simulink model "Pulse24Rectifier"  (R2023b)
settings: Solver=VariableStepAuto  StartTime=0.0  StopTime=0.1  RelTol=1e-3
undefined symbols (not defined in the file or in its folder): D1, D11, Delta
libraries: spsCurrentMeasurementLib x26, spsDiodeLib x24, spsVoltageMeasurementLib x4, spsACVoltageSourceLib x3, spsThreePhaseTransformerThreeWindingsLib x2, spsGroundLib x1, spsSeriesRLCBranchLib x1, spsZigzagPhaseShiftingTransformerLib x1, spspowerguiLib x1
settings Model: Creator=HP  LastModifiedBy=HP
settings SolverCC: ZeroCrossAlgorithm=Adaptive
settings DataIOCC: Refine=10
settings DebuggingCC: IgnoredZcDiagnostic=none

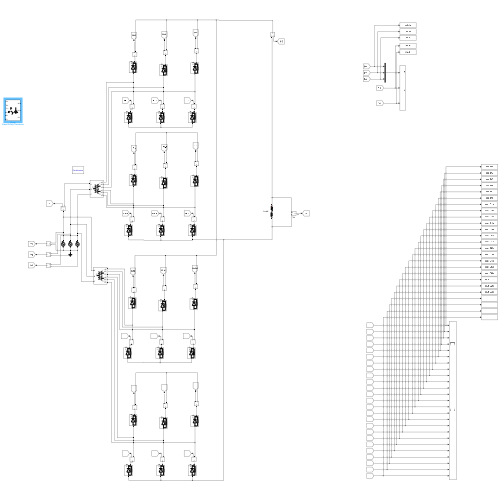
[thumbnail: Simulink's stored preview of the top-level diagram]
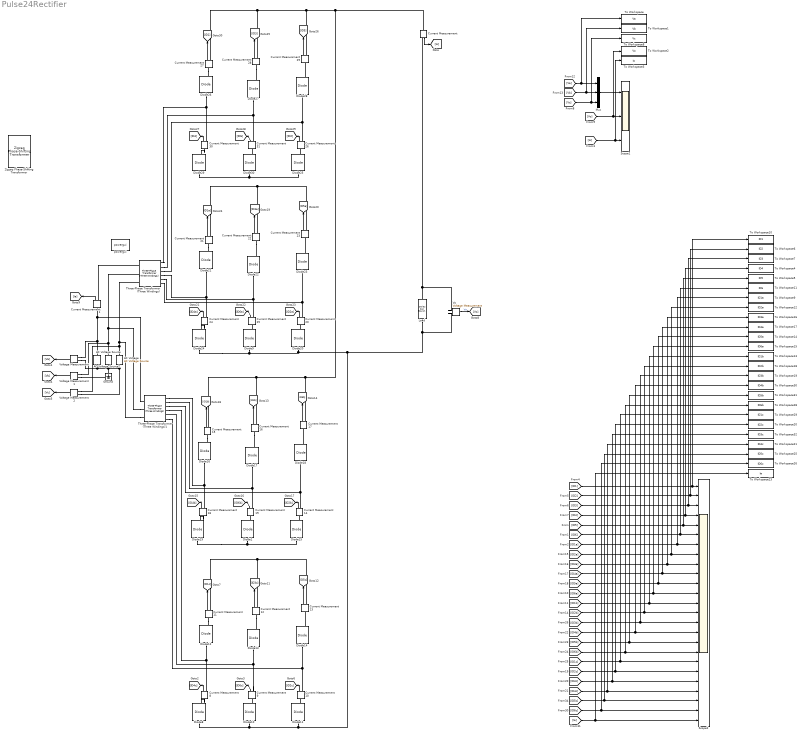
== system Pulse24Rectifier ==
  AC Voltage : spsACVoltageSourceLib/AC Voltage Source  Amplitude=480*sqrt(2)/sqrt(3)  Phase=120  Frequency=60  SampleTime=0  Measurements=None  BusType=swing  Pref=10e3  Qref=0  Qmin=-inf  Qmax=+inf
  AC Voltage Source : spsACVoltageSourceLib/AC Voltage Source  Amplitude=480*sqrt(2)/sqrt(3)  Phase=-120  Frequency=60  SampleTime=0  Measurements=None  BusType=swing  Pref=10e3  Qref=0  Qmin=-inf  Qmax=+inf
  AC Voltage Source2 : spsACVoltageSourceLib/AC Voltage Source  Amplitude=480*sqrt(2)/sqrt(3)  Phase=0  Frequency=60  SampleTime=0  Measurements=None  BusType=swing  Pref=10e3  Qref=0  Qmin=-inf  Qmax=+inf
  Current Measurement{,1,8..31} (26 alike) : spsCurrentMeasurementLib/Current Measurement  PhasorSimulation=off  OutputType=Complex  PSBequivalent=0
  Diode{1,8..30} (24 alike) : spsDiodeLib/Diode  Ron=0.001  Lon=0  Vf=0.8  IC=0  UseSnubber=0  Rs=500  Cs=250e-9  Measurements=on
  Ground : spsGroundLib/Ground  LConnTagsString=a
  Load : spsSeriesRLCBranchLib/Series RLC Branch  LConnTagsString=__new0  RConnTagsString=__new0  BranchType=RL  Resistance=11.08  Inductance=0.0224  SetiL0=off  InitialCurrent=0  Capacitance=1e-6  Setx0=off  InitialVoltage=0  Measurements=None
  Mux : Mux  Inputs=3
  Scope1 : Scope  NumInputPorts=3
  Scope2 : Scope  NumInputPorts=25
  Three-Phase Transformer (Three Windings) : spsThreePhaseTransformerThreeWindingsLib/Three-Phase Transformer (Three Windings)  Winding1Connection=Delta (D1)  Winding2Connection=Y  Winding3Connection=Delta (D11)  CoreType=Three single-phase transformers  SetSaturation=off  Hysteresis=off  DataFile='hysteresis'  SetInitialFlux=off  Measurements=None  UNITS=pu  NominalPower=[ 250e3 , 50 ]  Winding1=[ 300 , 0.002 , 0.08 ]  Winding2=[ 100 , 0.002 , 0.08 ]  Winding3=[ 100 , 0.002 , 0.08 ]  Rm=500  Lm=500  L0=0.5  Saturation=[ 0,0 ; 0.0024,1.2 ; 1.0,1.52 ]  InitialFluxes=[0.8 -0.8 0.7]  BreakLoop=off  DiscreteSolver=Trapezoidal iterative  DataType=off  TransfoNumber=1
      settings: LibrarySourceBlock=|
      | sps_lib/Power Grid Elements/Three-Phase
      | Transformer
      | (Three Windings)
  Three-Phase Transformer (Three Windings)1 : spsThreePhaseTransformerThreeWindingsLib/Three-Phase Transformer (Three Windings)  Winding1Connection=Delta (D1)  Winding2Connection=Y  Winding3Connection=Delta (D11)  CoreType=Three single-phase transformers  SetSaturation=off  Hysteresis=off  DataFile='hysteresis'  SetInitialFlux=off  Measurements=None  UNITS=pu  NominalPower=[ 250e3 , 50 ]  Winding1=[ 300 , 0.002 , 0.08 ]  Winding2=[ 100 , 0.002 , 0.08 ]  Winding3=[ 100 , 0.002 , 0.08 ]  Rm=500  Lm=500  L0=0.5  Saturation=[ 0,0 ; 0.0024,1.2 ; 1.0,1.52 ]  InitialFluxes=[0.8 -0.8 0.7]  BreakLoop=off  DiscreteSolver=Trapezoidal iterative  DataType=off  TransfoNumber=1
      settings: LibrarySourceBlock=|
      | sps_lib/Power Grid Elements/Three-Phase
      | Transformer
      | (Three Windings)
  To Workspace : ToWorkspace  VariableName=Va  SaveFormat=Timeseries  SampleTime=-1
  To Workspace1 : ToWorkspace  VariableName=Vb  SaveFormat=Timeseries  SampleTime=-1
  To Workspace10 : ToWorkspace  VariableName=ID1  SaveFormat=Timeseries  SampleTime=-1
  To Workspace11 : ToWorkspace  VariableName=ID6  SaveFormat=Timeseries  SampleTime=-1
  To Workspace12 : ToWorkspace  VariableName=ID2a  SaveFormat=Timeseries  SampleTime=-1
  To Workspace13 : ToWorkspace  VariableName=ID1b  SaveFormat=Timeseries  SampleTime=-1
  To Workspace14 : ToWorkspace  VariableName=ID5a  SaveFormat=Timeseries  SampleTime=-1
  To Workspace15 : ToWorkspace  VariableName=ID6a  SaveFormat=Timeseries  SampleTime=-1
  To Workspace16 : ToWorkspace  VariableName=ID3a  SaveFormat=Timeseries  SampleTime=-1
  To Workspace17 : ToWorkspace  VariableName=ID4a  SaveFormat=Timeseries  SampleTime=-1
  To Workspace18 : ToWorkspace  VariableName=ID2b  SaveFormat=Timeseries  SampleTime=-1
  To Workspace19 : ToWorkspace  VariableName=ID3b  SaveFormat=Timeseries  SampleTime=-1
  To Workspace2 : ToWorkspace  VariableName=Vo  SaveFormat=Timeseries  SampleTime=-1
  To Workspace20 : ToWorkspace  VariableName=ID2c  SaveFormat=Timeseries  SampleTime=-1
  To Workspace21 : ToWorkspace  VariableName=ID4c  SaveFormat=Timeseries  SampleTime=-1
  To Workspace23 : ToWorkspace  VariableName=Ia  SaveFormat=Timeseries  SampleTime=-1
  To Workspace25 : ToWorkspace  VariableName=ID5c  SaveFormat=Timeseries  SampleTime=-1
  To Workspace26 : ToWorkspace  VariableName=ID6c  SaveFormat=Timeseries  SampleTime=-1
  To Workspace28 : ToWorkspace  VariableName=ID6b  SaveFormat=Timeseries  SampleTime=-1
  To Workspace29 : ToWorkspace  VariableName=ID1c  SaveFormat=Timeseries  SampleTime=-1
  To Workspace3 : ToWorkspace  VariableName=Io  SaveFormat=Timeseries  SampleTime=-1
  To Workspace30 : ToWorkspace  VariableName=ID4b  SaveFormat=Timeseries  SampleTime=-1
  To Workspace31 : ToWorkspace  VariableName=ID5b  SaveFormat=Timeseries  SampleTime=-1
  To Workspace32 : ToWorkspace  VariableName=ID3c  SaveFormat=Timeseries  SampleTime=-1
  To Workspace4 : ToWorkspace  VariableName=ID4  SaveFormat=Timeseries  SampleTime=-1
  To Workspace5 : ToWorkspace  VariableName=ID5  SaveFormat=Timeseries  SampleTime=-1
  To Workspace6 : ToWorkspace  VariableName=ID2  SaveFormat=Timeseries  SampleTime=-1
  To Workspace7 : ToWorkspace  VariableName=ID3  SaveFormat=Timeseries  SampleTime=-1
  To Workspace8 : ToWorkspace  VariableName=Vc  SaveFormat=Timeseries  SampleTime=-1
  To Workspace9 : ToWorkspace  VariableName=ID1a  SaveFormat=Timeseries  SampleTime=-1
  Vo : spsVoltageMeasurementLib/Voltage Measurement  PhasorSimulation=off  OutputType=Complex  PSBequivalent=0
  Voltage Measurement : spsVoltageMeasurementLib/Voltage Measurement  PhasorSimulation=off  OutputType=Complex  PSBequivalent=0
  Voltage Measurement1 : spsVoltageMeasurementLib/Voltage Measurement  PhasorSimulation=off  OutputType=Complex  PSBequivalent=0
  Voltage Measurement2 : spsVoltageMeasurementLib/Voltage Measurement  PhasorSimulation=off  OutputType=Complex  PSBequivalent=0
  Zigzag Phase-Shifting Transformer : spsZigzagPhaseShiftingTransformerLib/Zigzag Phase-Shifting Transformer  SecondaryConnection=Yg  SetSaturation=off  SetInitialFlux=off  Measurements=None  UNITS=pu  NominalPower=[ 100e6 60]  PrimaryVoltage=10e3  SecondaryVoltage="[ 30e3  +15]"  Winding1=[ 0.002 0.08 ]  Winding2="[ 0.002  0.08 ]"  Winding3=[ 0.002 0.08 ]  RmLm=[ 500 500 ]  Rm=500  Saturation=[ 0,0 ; 0.0024,1.2 ; 1.0,1.52 ]  InitialFluxes=[0,0,0]  BreakLoop=off  DiscreteSolver=Trapezoidal iterative  DataType=off
      settings: LibrarySourceBlock=|
      | sps_lib/Power Grid Elements/Zigzag
      | Phase-Shifting Transformer
  powergui : spspowerguiLib/powergui  Priority=1  SimulationMode=Continuous  SampleTime=50e-6  frequency=60  Iterations=50  frequencyindice=60  Pbase=100e6  ErrMax=1e-4  UnitsV=kV  UnitsW=MW  buscounter=0  FunctionMessages=off  echomessages=off  EnableUseOfTLC=off  CurrentSourceSwitches=off  DisableSnubberDevices=off  DisableRonSwitches=off  DisableVfSwitches=off  DisplayEquations=off  AutomaticDiscreteSolvers=off  SolverType=Tustin/Backward Euler (TBE)  Interpol=off  ExternalGateDelay=off  methode=off  Ts=0  x0status=blocks  SPID=off  SwTol=0  HookPort=off  NonlinearTolerance=1e-4  nMaxIteration=100  ContinueOnMaxIteration=off  RestoreLinks=warning  ResistiveCurrentMeasurement=off  Frange=[0:2:500]  Ylog=off  Xlog=on  ShowGrid=off  save=off  variable=ZData  structure=0  ZoomFFT=on  StartTime=0.0  cycles=1  DisplayStyle=1  fundamental=60  FreqAxis=off  MaxFrequency=1000  frequencyindicesteady=1  RmsSteady=1  display=off
  wires:
  Vo/1 -> [Vo]  "Vo"
  Current Measurement8/1 -> [ID4c]
  Current Measurement9/1 -> [ID6c]
  Current Measurement10/1 -> [ID2c]
  Current Measurement11/1 -> [ID1c]
  Current Measurement12/1 -> [ID3c]
  Current Measurement13/1 -> [ID5c]
  Current Measurement17/1 -> [ID5b]
  Current Measurement16/1 -> [ID3b]
  Current Measurement15/1 -> [ID1b]
  Current Measurement14/1 -> [ID2b]
  Current Measurement19/1 -> [ID6b]
  Current Measurement18/1 -> [ID4b]
  Current Measurement24/1 -> [ID4a]
  Current Measurement25/1 -> [ID6a]
  Current Measurement20/1 -> [ID2a]
  Current Measurement21/1 -> [ID1a]
  Current Measurement22/1 -> [ID3a]
  Current Measurement23/1 -> [ID5a]
  Current Measurement29/1 -> [ID5]
  Current Measurement28/1 -> [ID3]
  Current Measurement27/1 -> [ID1]
  Current Measurement26/1 -> [ID2]
  Current Measurement31/1 -> [ID6]
  Current Measurement30/1 -> [ID4]
  Current Measurement/1 -> [Io]
  Voltage Measurement1/1 -> [Vb]
  Voltage Measurement/1 -> [Va]
  Voltage Measurement2/1 -> [Vc]
  [ID4] -> To Workspace4/1, Scope2/4
  [ID6] -> Scope2/6, To Workspace11/1
  [ID1] -> To Workspace10/1, Scope2/1
  [Io] -> To Workspace3/1, Scope1/3
  [Vo] -> To Workspace2/1, Scope1/2
  Mux/1 -> Scope1/1
  [ID5] -> Scope2/5, To Workspace5/1
  [ID2] -> To Workspace6/1, Scope2/2
  [ID3] -> To Workspace7/1, Scope2/3
  [Vc] -> To Workspace8/1, Mux/3
  [Va] -> To Workspace/1, Mux/1
  [ID1a] -> Scope2/7, To Workspace9/1
  [Vb] -> To Workspace1/1, Mux/2
  [Ia] -> To Workspace23/1, Scope2/25
  [ID6c] -> To Workspace26/1, Scope2/24
  [ID5c] -> To Workspace25/1, Scope2/23
  [ID4c] -> To Workspace21/1, Scope2/22
  Current Measurement1/1 -> [Ia]
  [ID2a] -> To Workspace12/1, Scope2/8
  [ID3a] -> To Workspace16/1, Scope2/9
  [ID4a] -> To Workspace17/1, Scope2/10
  [ID5a] -> To Workspace14/1, Scope2/11
  [ID6a] -> To Workspace15/1, Scope2/12
  [ID1b] -> To Workspace13/1, Scope2/13
  [ID2b] -> To Workspace18/1, Scope2/14
  [ID3b] -> To Workspace19/1, Scope2/15
  [ID4b] -> To Workspace30/1, Scope2/16
  [ID5b] -> To Workspace31/1, Scope2/17
  [ID6b] -> To Workspace28/1, Scope2/18
  [ID1c] -> To Workspace29/1, Scope2/19
  [ID2c] -> To Workspace20/1, Scope2/20
  [ID3c] -> To Workspace32/1, Scope2/21
  connections:
  Three-Phase Transformer (Three Windings)1/LConn1 -- AC Voltage Source2/RConn1 -- Voltage Measurement/LConn1 -- Current Measurement1/LConn1
  Three-Phase Transformer (Three Windings)1/LConn2 -- AC Voltage Source/RConn1 -- Voltage Measurement1/LConn1 -- Three-Phase Transformer (Three Windings)/LConn2
  Three-Phase Transformer (Three Windings)1/LConn3 -- AC Voltage/RConn1 -- Voltage Measurement2/LConn1 -- Three-Phase Transformer (Three Windings)/LConn3
  Three-Phase Transformer (Three Windings)1/RConn6 -- Current Measurement10/RConn1 -- Diode14/LConn1
  Current Measurement9/RConn1 -- Three-Phase Transformer (Three Windings)1/RConn5 -- Diode13/LConn1
  Three-Phase Transformer (Three Windings)1/RConn4 -- Diode12/LConn1 -- Current Measurement8/RConn1
  AC Voltage Source/LConn1 -- AC Voltage Source2/LConn1 -- Voltage Measurement/LConn2 -- Voltage Measurement2/LConn2 -- AC Voltage/LConn1 -- Ground/LConn1 -- Voltage Measurement1/LConn2
  Current Measurement8/LConn1 -- Diode8/RConn1
  Diode10/RConn1 -- Current Measurement9/LConn1
  Diode11/RConn1 -- Current Measurement10/LConn1
  Current Measurement11/LConn1 -- Diode12/RConn1
  Current Measurement12/LConn1 -- Diode13/RConn1
  Diode14/RConn1 -- Current Measurement13/LConn1
  Current Measurement12/RConn1 -- Current Measurement13/RConn1 -- Current Measurement11/RConn1
  Diode15/LConn1 -- Diode19/LConn1 -- Diode1/LConn1
  Current Measurement14/RConn1 -- Diode18/LConn1 -- Three-Phase Transformer (Three Windings)1/RConn3
  Diode17/LConn1 -- Three-Phase Transformer (Three Windings)1/RConn2 -- Current Measurement19/RConn1
  Diode16/LConn1 -- Three-Phase Transformer (Three Windings)1/RConn1 -- Current Measurement18/RConn1
  Diode18/RConn1 -- Current Measurement17/LConn1
  Current Measurement16/LConn1 -- Diode17/RConn1
  Diode1/RConn1 -- Current Measurement19/LConn1
  Current Measurement18/LConn1 -- Diode19/RConn1
  Current Measurement15/LConn1 -- Diode16/RConn1
  Diode15/RConn1 -- Current Measurement14/LConn1
  Diode10/LConn1 -- Vo/LConn2 -- Load/RConn1 -- Diode9/LConn1 -- Diode24/LConn1 -- Diode20/LConn1 -- Diode11/LConn1 -- Diode8/LConn1
  Current Measurement20/RConn1 -- Diode23/LConn1 -- Three-Phase Transformer (Three Windings)/RConn6
  Diode22/LConn1 -- Three-Phase Transformer (Three Windings)/RConn5 -- Current Measurement25/RConn1
  Diode21/LConn1 -- Three-Phase Transformer (Three Windings)/RConn4 -- Current Measurement24/RConn1
  Current Measurement23/RConn1 -- Current Measurement22/RConn1 -- Current Measurement21/RConn1
  Current Measurement21/LConn1 -- Diode21/RConn1
  Current Measurement24/LConn1 -- Diode24/RConn1
  Diode20/RConn1 -- Current Measurement20/LConn1
  Diode23/RConn1 -- Current Measurement23/LConn1
  Current Measurement22/LConn1 -- Diode22/RConn1
  Diode9/RConn1 -- Current Measurement25/LConn1
  Diode30/LConn1 -- Diode25/LConn1 -- Diode29/LConn1
  Current Measurement26/RConn1 -- Three-Phase Transformer (Three Windings)/RConn3 -- Diode28/LConn1
  Diode27/LConn1 -- Three-Phase Transformer (Three Windings)/RConn2 -- Current Measurement31/RConn1
  Diode26/LConn1 -- Three-Phase Transformer (Three Windings)/RConn1 -- Current Measurement30/RConn1
  Current Measurement17/RConn1 -- Current Measurement28/RConn1 -- Current Measurement27/RConn1 -- Current Measurement29/RConn1 -- Current Measurement/LConn1 -- Current Measurement15/RConn1 -- Current Measurement16/RConn1
  Diode30/RConn1 -- Current Measurement31/LConn1
  Current Measurement28/LConn1 -- Diode27/RConn1
  Diode28/RConn1 -- Current Measurement29/LConn1
  Current Measurement27/LConn1 -- Diode26/RConn1
  Current Measurement30/LConn1 -- Diode29/RConn1
  Diode25/RConn1 -- Current Measurement26/LConn1
  Vo/LConn1 -- Load/LConn1 -- Current Measurement/RConn1
  Current Measurement1/RConn1 -- Three-Phase Transformer (Three Windings)/LConn1
